simulink model "Flight_Simulation"  (R2021b)
settings: Solver=ode4  StartTime=0.0  StopTime=20  FixedStep=Settings.Simulation.step_size  RelTol=1e-3  EnableMultiTasking=on
undefined symbols (not defined in the file or in its folder): AeroCoeff, Aircraft, ControlGains, dLEF, Environment, F, Light, MIL, Settings, Trim, trim_control, trim_state, trim_thrust
libraries: simulink x19, simulink_extras x14, slpidlib x2, aerolibfltsims x2, aerolibwind2 x1, vrlib x1
(part 3 of 5)

== system Flight_Simulation/Environment_Subsystems/Wind_Input/Bypass for TrimAndLin ==
  note: No time variant wind for TrimAndLin
  Wind_BUS : Inport
  Flag_Settings_BUS : Inport  Port=2
  Bus Creator : BusCreator  Inputs=3
  Bus Selector : BusSelector  OutputSignals=Linearization_Flag,Trim_Flag
  Bypass for TrimAndLin : Switch  Criteria=u2 > Threshold
  Constant : Constant  Value=0
  Constant1 : Constant  Value=0
  Constant2 : Constant  Value=0
  Demux : Demux  Outputs=3
  Logical Operator : Logic  Operator=NOR  AllPortsSameDT=off  OutDataTypeStr=boolean
  Mux1 : Mux  Inputs=3
  Wind_Vel : Outport
  wires:
  Bus Selector/2 -> Logical Operator/2  "<Trim_Flag>"
  Bus Selector/1 -> Logical Operator/1  "<Linearization_Flag>"
  Logical Operator/1 -> Bypass for TrimAndLin/2
  Flag_Settings_BUS/1 -> Bus Selector/1
  Bus Creator/1 -> Wind_Vel/1  "Wind_Vel_UVWe_m/s"
  Demux/1 -> Bus Creator/1  "u_wind_m/s"
  Demux/2 -> Bus Creator/2  "v_wind_m/s"
  Demux/3 -> Bus Creator/3  "w_wind_m/s"
  Bypass for TrimAndLin/1 -> Demux/1
  Wind_BUS/1 -> Bypass for TrimAndLin/1
  Constant1/1 -> Mux1/1  "u_wind_m/s"
  Constant/1 -> Mux1/2  "v_wind_m/s"
  Constant2/1 -> Mux1/3  "w_wind_m/s"
  Mux1/1 -> Bypass for TrimAndLin/3

== system Flight_Simulation/Environment_Subsystems/Wind_Input/Calc_Vel_aero_alpha_beta ==
  Vel_U_V_W_BUS : Inport
  Add : Sum  Inputs=+++
  Atan : Trigonometry  Operator=atan
  Atan1 : Trigonometry  Operator=atan
  Bus Creator : BusCreator  Inputs=3
  Bus Selector : BusSelector  OutputSignals=U_aero_m/s,V_aero_m/s,W_aero_m/s
  Divide : Product  Inputs=*/
  Divide1 : Product  Inputs=*/
  Sqrt : Sqrt  SaturateOnIntegerOverflow=on
  Square : Math  Operator=square  SaturateOnIntegerOverflow=on
  Square1 : Math  Operator=square  SaturateOnIntegerOverflow=on
  Square2 : Math  Operator=square  SaturateOnIntegerOverflow=on
  Vel_aero_alpha_beta_BUS : Outport
  wires:
  Vel_U_V_W_BUS/1 -> Bus Selector/1
  Bus Creator/1 -> Vel_aero_alpha_beta_BUS/1  "Vel_aero_V_alpha_beta"
  Sqrt/1 -> Bus Creator/1  "v_m/s"
  Atan/1 -> Bus Creator/2  "alpha_rad"
  Atan1/1 -> Bus Creator/3  "beta_rad"
  Bus Selector/1 -> Divide1/2, Divide/2, Square/1  "<U_aero_m/s>"
  Bus Selector/2 -> Square1/1, Divide1/1  "<V_aero_m/s>"
  Bus Selector/3 -> Divide/1, Square2/1  "<W_aero_m/s>"
  Add/1 -> Sqrt/1
  Square2/1 -> Add/3
  Square1/1 -> Add/2
  Square/1 -> Add/1
  Divide/1 -> Atan/1
  Divide1/1 -> Atan1/1

== system Flight_Simulation/Environment_Subsystems/Wind_Model/Gust_model_(1-cos) ==
  note: To stop the "distance traveled
      | through the gust counter"
  Atmosphere_BUS : Inport
  FlightProfileAlleviationFactor_Fg : Inport  Port=2
  altitude_m : Inport  Port=3
  v_m/s : Inport  Port=4
  1-cos_gust_flg : Step  Time=Environment.gust.steptimes  After=Environment.gust.flags  SampleTime=0
  Abs1 : Abs
  Distance traveled through the gust : Subsystem
  Gust parameters : Subsystem
  Gust velocity (1-cos) : Subsystem
      mask Display: image('1-cos-gust.png'); % Use "Edit Image" on toolstrip to change.
  Sum1 : Sum  Inputs=|+-
  reset flags after gust : Subsystem
  u_wind_m/s : Outport
  v_wind_m/s : Outport  Port=2
  w_wind_m/s : Outport  Port=3
  wires:
  Sum1/1 -> Distance traveled through the gust/2(gust_flgs)  "gust_flgs"
  reset flags after gust/1(reset_flgs) -> Sum1/2
  1-cos_gust_flg/1 -> Abs1/1, Gust velocity (1-cos)/4(Sign_Input)  "Sign_carry"
  altitude_m/1 -> Gust parameters/3(altitude)
  Gust parameters/1(gust_gradient_length) -> Gust velocity (1-cos)/1(gust_gradient_length)
  Abs1/1 -> Sum1/1
  Gust parameters/2(gust_amplitudes) -> Gust velocity (1-cos)/2(gust_amplitudes)
  Distance traveled through the gust/1(distance_traveled) -> Gust velocity (1-cos)/3(distance_traveled)  "distance_traveled_xyz"
  Gust velocity (1-cos)/2(Gust_Vel_V_m/s) -> reset flags after gust/2(gust_v), v_wind_m/s/1  "v_wind_m/s"
  v_m/s/1 -> Distance traveled through the gust/1(v_m/s)
  FlightProfileAlleviationFactor_Fg/1 -> Gust parameters/2(F_g)
  Gust velocity (1-cos)/1(Gust_Vel_U_m/s) -> reset flags after gust/1(gust_u), u_wind_m/s/1  "u_wind_m/s"
  Gust velocity (1-cos)/3(Gust_Vel_W_m/s) -> reset flags after gust/3(gust_w), w_wind_m/s/1  "w_wind_m/s"
  Atmosphere_BUS/1 -> Gust parameters/1(Atmosphere_BUS)

== system Flight_Simulation/Non-linear_Plant/6DOF_Equations/Acceleration_nx_ny_nz_Calculation ==
  Vel_U_V_W_dot_BUS : Inport
  States_BUS : Inport  Port=2
  Gravity_BUS : Inport  Port=3
  Bus Creator : BusCreator  Inputs=3
  nx_cg : Subsystem
  ny_cg : Subsystem
  nz_cg : Subsystem
  Acc_nx_ny_nz_BUS : Outport
  wires:
  States_BUS/1 -> nx_cg/1(States_BUS), nz_cg/1(States_BUS), ny_cg/1(States_BUS)
  Vel_U_V_W_dot_BUS/1 -> nx_cg/2(Vel_U_V_W_dot_BUS), nz_cg/2(Vel_U_V_W_dot_BUS), ny_cg/2(Vel_U_V_W_dot_BUS)
  Gravity_BUS/1 -> nx_cg/3(Gravity), nz_cg/3(Gravity), ny_cg/3(Gravity)
  Bus Creator/1 -> Acc_nx_ny_nz_BUS/1
  nx_cg/1(n_x_cg) -> Bus Creator/1
  ny_cg/1(n_y_cg) -> Bus Creator/2
  nz_cg/1(n_z_cg) -> Bus Creator/3

== system Flight_Simulation/Non-linear_Plant/6DOF_Equations/Attitude_Differential_Equations ==
  States_BUS : Inport
  Bus Creator : BusCreator  Inputs=3
  Bus Selector : BusSelector  OutputSignals=Angles_phi_theta_psi,Rates_p_q_r
  Bus Selector1 : BusSelector  OutputSignals=phi_rad,theta_rad,psi_rad
  Bus Selector2 : BusSelector  OutputSignals=p_rad/s,q_rad/s,r_rad/s
  phi_dot : Subsystem
  psi_dot : Subsystem
  theta_dot : Subsystem
  Attitude_dot_BUS : Outport
  wires:
  States_BUS/1 -> Bus Selector/1
  Bus Selector/1 -> Bus Selector1/1  "<Angles_phi_theta_psi>"
  Bus Selector/2 -> Bus Selector2/1  "<Rates_p_q_r>"
  Bus Creator/1 -> Attitude_dot_BUS/1  "Angles_dot_phi_theta_psi"
  Bus Selector1/1 -> phi_dot/1(phi), theta_dot/1(phi), psi_dot/1(phi)  "<phi_rad>"
  Bus Selector1/2 -> phi_dot/2(theta), theta_dot/2(theta), psi_dot/2(theta)  "<theta_rad>"
  Bus Selector1/3 -> phi_dot/3(psi), psi_dot/3(psi), theta_dot/3(psi)  "<psi_rad>"
  Bus Selector2/1 -> phi_dot/4(p), psi_dot/4(p), theta_dot/4(p)  "<p_rad/s>"
  Bus Selector2/2 -> phi_dot/5(q), psi_dot/5(q), theta_dot/5(q)  "<q_rad/s>"
  Bus Selector2/3 -> phi_dot/6(r), psi_dot/6(r), theta_dot/6(r)  "<r_rad/s>"
  phi_dot/1(phi_dot_rad/s) -> Bus Creator/1
  theta_dot/1(theta_dot_rad/s) -> Bus Creator/2
  psi_dot/1(psi_dot_rad/s) -> Bus Creator/3

== system Flight_Simulation/Non-linear_Plant/6DOF_Equations/Position_Differential_Equations ==
  Earth_Model_BUS : Inport
  States_BUS : Inport  Port=2
  Bus Creator : BusCreator  Inputs=3
  Bus Creator2 : BusCreator  Inputs=2
  Bus Selector : BusSelector  OutputSignals=Angles_phi_theta_psi
  Bus Selector1 : BusSelector  OutputSignals=U_m/s,V_m/s,W_m/s
  Bus Selector2 : BusSelector  OutputSignals=Pos_WGS84
  Bus Selector3 : BusSelector  OutputSignals=phi_rad,theta_rad,psi_rad
  Bus Selector4 : BusSelector  OutputSignals=Vel_U_V_W_body
  Calculate_alt_position_dot1 : Subsystem
  Calculate_east_position_dot : Subsystem
  Calculate_north_position_dot : Subsystem
  Position_dot_WGS84 : Subsystem
  Position_dot_BUS : Outport
  wires:
  Bus Creator/1 -> Bus Creator2/1  "Position_dot_north_east_alt"
  Bus Selector/1 -> Bus Selector3/1  "<Angles_phi_theta_psi>"
  Bus Selector1/1 -> Calculate_north_position_dot/1(U), Calculate_east_position_dot/1(U), Calculate_alt_position_dot1/1(U)  "<U_m/s>"
  Bus Selector1/2 -> Calculate_north_position_dot/2(V), Calculate_alt_position_dot1/2(V), Calculate_east_position_dot/2(V)  "<V_m/s>"
  Bus Selector1/3 -> Calculate_north_position_dot/3(W), Calculate_alt_position_dot1/3(W), Calculate_east_position_dot/3(W)  "<W_m/s>"
  Bus Selector3/1 -> Calculate_north_position_dot/4(phi), Calculate_alt_position_dot1/4(phi), Calculate_east_position_dot/4(phi)  "<phi_rad>"
  Bus Selector3/2 -> Calculate_alt_position_dot1/5(theta), Calculate_east_position_dot/5(theta), Calculate_north_position_dot/5(theta)  "<theta_rad>"
  Bus Selector3/3 -> Calculate_alt_position_dot1/6(psi), Calculate_east_position_dot/6(psi), Calculate_north_position_dot/6(psi)  "<psi_rad>"
  Calculate_north_position_dot/1(north_pos_dot) -> Position_dot_WGS84/1(U_earth), Bus Creator/1
  Calculate_east_position_dot/1(east_pos_dot) -> Position_dot_WGS84/2(V_earth), Bus Creator/2
  Calculate_alt_position_dot1/1(alt_dot) -> Position_dot_WGS84/3(alt_dot), Bus Creator/3
  Earth_Model_BUS/1 -> Position_dot_WGS84/5(Earth_Model_BUS)
  Position_dot_WGS84/1(Pos_WGS84_dot_BUS) -> Bus Creator2/2
  Bus Creator2/1 -> Position_dot_BUS/1  "Position_dot_BUS"
  Bus Selector2/1 -> Position_dot_WGS84/4(Pos_WGS84)  "<Pos_WGS84>"
  States_BUS/1 -> Bus Selector4/1, Bus Selector2/1, Bus Selector/1
  Bus Selector4/1 -> Bus Selector1/1  "<Vel_U_V_W_body>"

== system Flight_Simulation/Non-linear_Plant/6DOF_Equations/Rotation_Differential_Equation ==
  Aircraft_Constants_BUS : Inport
  Engine_BUS : Inport  Port=2
  States_BUS : Inport  Port=3
  Moments_total_BUS : Inport  Port=4
  Bus Creator1 : BusCreator  Inputs=3
  Inertia_Denominator_Calculation : Subsystem
  p_dot_Calculation : Subsystem
  q_dot_Calculation : Subsystem
  r_dot_Calculation : Subsystem
  Rates_dot_p_q_r : Outport
  wires:
  Aircraft_Constants_BUS/1 -> r_dot_Calculation/3(Aircraft_Constants_BUS), p_dot_Calculation/2(Aircraft_Constants_BUS), q_dot_Calculation/2(Aircraft_Constants_BUS), Inertia_Denominator_Calculation/1(Aircraft_Constants_BUS)
  States_BUS/1 -> r_dot_Calculation/2(States_BUS), p_dot_Calculation/3(States_BUS), q_dot_Calculation/1(States_BUS)
  Inertia_Denominator_Calculation/1(Inertia_Denominator) -> r_dot_Calculation/1(Inertia_Denominator), p_dot_Calculation/4(Inertia_Denominator)
  Moments_total_BUS/1 -> r_dot_Calculation/4(Moments_total_BUS), p_dot_Calculation/1(Moments_total_BUS), q_dot_Calculation/3(Moments_total_BUS)  "Moments_total_BUS"
  p_dot_Calculation/1(p_dot) -> Bus Creator1/1
  q_dot_Calculation/1(q_dot) -> Bus Creator1/2
  Bus Creator1/1 -> Rates_dot_p_q_r/1  "Rates_dot_p_q_r"
  r_dot_Calculation/1(r_dot) -> Bus Creator1/3
  Engine_BUS/1 -> q_dot_Calculation/4(Engine_BUS)

== system Flight_Simulation/Non-linear_Plant/6DOF_Equations/Translation_UVW_Differential_Equations ==
  States_BUS : Inport
  Forces_total_BUS : Inport  Port=2
  Engine_BUS : Inport  Port=3
  Aircraft_Constants_BUS : Inport  Port=4
  Gravity_BUS : Inport  Port=5
  Bus Creator : BusCreator  Inputs=3
  U_dot : Subsystem
  V_dot : Subsystem
  W_dot : Subsystem
  Vel_U_V_W_body_dot_BUS : Outport
  wires:
  Bus Creator/1 -> Vel_U_V_W_body_dot_BUS/1  "Vel_U_V_W_body_dot_BUS"
  U_dot/1(U_dot) -> Bus Creator/1
  States_BUS/1 -> U_dot/1(States_BUS), V_dot/1(States_BUS), W_dot/1(States_BUS)
  Forces_total_BUS/1 -> W_dot/2(Force_Coeff_BUS), U_dot/2(Forces_total_BUS), V_dot/2(Forces_total_BUS)
  Aircraft_Constants_BUS/1 -> U_dot/3(Aircraft_Constants_BUS), W_dot/3(Aircraft_Constants_BUS), V_dot/3(Aircraft_Constants_BUS1)
  Gravity_BUS/1 -> W_dot/4(Gravity_BUS), V_dot/4(Gravity_BUS), U_dot/4(Gravity_BUS)
  Engine_BUS/1 -> U_dot/5(Engine_BUS)
  V_dot/1(V_dot) -> Bus Creator/2
  W_dot/1(W_dot) -> Bus Creator/3

== system Flight_Simulation/Non-linear_Plant/Actuator_Models/Aileron Actuator ==
  note: Mustn't change the name of integrator representing the position
      | xxx_pos_int as this will interfere with the trim and lin routine
  Aileron_cmd_deg : Inport
  Control_Surface_Const_BUS : Inport  Port=2
  Aileron_init_deg : Inport  Port=3
  Ail_pos_int : Integrator  InitialConditionSource=external  InitialCondition=trim_control(2)  UpperSaturationLimit=21.5  LowerSaturationLimit=-21.5
  Bus Selector : BusSelector  OutputSignals=Aileron_BUS.Ail_pos_max_deg,Aileron_BUS.Ail_pos_min_deg,Aileron_BUS.Ail_rate_max_degPs,Aileron_BUS.Ail_rate_min_degPs,Aileron_BUS.Ail_lag_s
  Command Saturation : simulink/Discontinuities/Saturation Dynamic  OutMin=[]  OutMax=[]  OutDataTypeStr=Inherit: Same as second input  OutDataType=fixdt(1, 16)  OutScaling=2^-10  DoSatur=off
  Divide : Product  Inputs=/*
  Rate Saturation : simulink/Discontinuities/Saturation Dynamic  OutMin=[]  OutMax=[]  OutDataTypeStr=Inherit: Same as second input  OutDataType=fixdt(1, 16)  OutScaling=2^-10  DoSatur=off
  Sum : Sum  Inputs=|+-  InputSameDT=on  SaturateOnIntegerOverflow=on  OutDataTypeStr=Inherit: Same as first input
  Aileron_act_deg : Outport
  wires:
  Rate Saturation/1 -> Ail_pos_int/1
  Aileron_cmd_deg/1 -> Command Saturation/2
  Aileron_init_deg/1 -> Ail_pos_int/2
  Bus Selector/3 -> Rate Saturation/1  "<Ail_rate_max_degPs>"
  Bus Selector/5 -> Divide/1  "<Ail_lag_s>"
  Bus Selector/4 -> Rate Saturation/3  "<Ail_rate_min_degPs>"
  Control_Surface_Const_BUS/1 -> Bus Selector/1
  Divide/1 -> Rate Saturation/2
  Bus Selector/1 -> Command Saturation/1  "<Ail_pos_max_deg>"
  Bus Selector/2 -> Command Saturation/3  "<Ail_pos_min_deg>"
  Command Saturation/1 -> Sum/1
  Sum/1 -> Divide/2
  Ail_pos_int/1 -> Aileron_act_deg/1, Sum/2

== system Flight_Simulation/Non-linear_Plant/Actuator_Models/Elevator Actuator ==
  note: Mustn't change the name of integrator representing the position
      | xxx_pos_int as this will interfere with the trim and lin routine
  Elevator_cmd_deg : Inport
  Control_Surface_Const_BUS : Inport  Port=2
  Elevator_init_deg : Inport  Port=3
  Bus Selector : BusSelector  OutputSignals=Elevator_BUS.Elev_pos_max_deg,Elevator_BUS.Elev_pos_min_deg,Elevator_BUS.Elev_rate_max_degPs,Elevator_BUS.Elev_rate_min_degPs,Elevator_BUS.Elev_lag_s
  Command Saturation : simulink/Discontinuities/Saturation Dynamic  OutMin=[]  OutMax=[]  OutDataTypeStr=Inherit: Same as second input  OutDataType=fixdt(1, 16)  OutScaling=2^-10  DoSatur=off
  Divide : Product  Inputs=/*
  Elev_pos_int : Integrator  InitialConditionSource=external  InitialCondition=trim_control(1)  UpperSaturationLimit=25  LowerSaturationLimit=-25
  Rate Saturation : simulink/Discontinuities/Saturation Dynamic  OutMin=[]  OutMax=[]  OutDataTypeStr=Inherit: Same as second input  OutDataType=fixdt(1, 16)  OutScaling=2^-10  DoSatur=off
  Sum : Sum  Inputs=|+-  InputSameDT=on  SaturateOnIntegerOverflow=on  OutDataTypeStr=Inherit: Same as first input
  Elevator_act_deg : Outport
  wires:
  Rate Saturation/1 -> Elev_pos_int/1
  Divide/1 -> Rate Saturation/2
  Sum/1 -> Divide/2
  Command Saturation/1 -> Sum/1
  Elevator_cmd_deg/1 -> Command Saturation/2
  Elevator_init_deg/1 -> Elev_pos_int/2
  Control_Surface_Const_BUS/1 -> Bus Selector/1
  Bus Selector/1 -> Command Saturation/1  "<Elev_pos_max_deg>"
  Bus Selector/2 -> Command Saturation/3  "<Elev_pos_min_deg>"
  Bus Selector/3 -> Rate Saturation/1  "<Elev_rate_max_degPs>"
  Bus Selector/4 -> Rate Saturation/3  "<Elev_rate_min_degPs>"
  Bus Selector/5 -> Divide/1  "<Elev_lag_s>"
  Elev_pos_int/1 -> Elevator_act_deg/1, Sum/2

== system Flight_Simulation/Non-linear_Plant/Actuator_Models/Leading Edge Flap ==
  note: initial state was:
      | -trim_state(8)*180/pi /// -alpha*180/pi
      |
      | set to 0 now, cause leading edge flap is not in use
      | change that to make the system more efficient
  note: see NASA Technical Paper 1538, p34
  note: Initialize LF_state with -alpha0 value in degrees!!!!
  Atmosphere_BUS : Inport
  States_BUS : Inport  Port=2
  Bus Selector1 : BusSelector  OutputSignals=alpha_rad
  Bus Selector2 : BusSelector  OutputSignals=Vel_aero_V_alpha_beta
  Bus Selector3 : BusSelector  OutputSignals=q_bar_Pa,p_static_Pa
  Divide : Product  Inputs=*/
  Gain : Gain  Gain=2  SaturateOnIntegerOverflow=on  OutDataTypeStr=Inherit: Same as input  ParamDataTypeStr=Inherit: Same as input
  Gain1 : Gain  Gain=7.25  SaturateOnIntegerOverflow=on  OutDataTypeStr=Inherit: Same as input  ParamDataTypeStr=Inherit: Same as input
  Gain2 : Gain  Gain=1.38  SaturateOnIntegerOverflow=on  OutDataTypeStr=Inherit: Same as input  ParamDataTypeStr=Inherit: Same as input
  LEF Actuator : Subsystem
  LEF deflection : ToWorkspace  Commented=on  VariableName=d_LF  SampleTime=-1
      settings: Decimation=100
  LF_state : Integrator
  Sum : Sum  Inputs=-|+|+  InputSameDT=on  SaturateOnIntegerOverflow=on  OutDataTypeStr=Inherit: Same as first input
  Sum1 : Sum  Inputs=|+-  InputSameDT=on  SaturateOnIntegerOverflow=on  OutDataTypeStr=Inherit: Same as first input
  Sum2 : Sum  Inputs=++|  InputSameDT=on  SaturateOnIntegerOverflow=on  OutDataTypeStr=Inherit: Same as first input
  coeff1 : Constant  Value=1.45
  r2d1 : Gain  Gain=180/pi  SaturateOnIntegerOverflow=on  OutDataTypeStr=Inherit: Same as input  ParamDataTypeStr=Inherit: Same as input
  r2d6 : Gain  Gain=9.05  SaturateOnIntegerOverflow=on  OutDataTypeStr=Inherit: Same as input  ParamDataTypeStr=Inherit: Same as input
  LE_Flap_deg : Outport
  wires:
  LEF Actuator/1(Out1) -> LEF deflection/1, LE_Flap_deg/1
  Sum/1 -> LEF Actuator/1(In1)
  States_BUS/1 -> Bus Selector2/1
  Sum1/1 -> Gain1/1
  Gain1/1 -> LF_state/1
  Gain/1 -> Sum2/1
  Gain2/1 -> Sum/2
  coeff1/1 -> Sum/3
  Sum2/1 -> Sum1/2, Gain2/1
  LF_state/1 -> Sum2/2
  r2d1/1 -> Sum1/1, Gain/1  "alpha"
  Divide/1 -> r2d6/1
  r2d6/1 -> Sum/1
  Bus Selector2/1 -> Bus Selector1/1  "<Vel_aero_V_alpha_beta>"
  Bus Selector1/1 -> r2d1/1  "<alpha_rad>"
  Atmosphere_BUS/1 -> Bus Selector3/1
  Bus Selector3/1 -> Divide/1  "<q_bar_Pa>"
  Bus Selector3/2 -> Divide/2  "<p_static_Pa>"

== system Flight_Simulation/Non-linear_Plant/Actuator_Models/Rudder Actuator ==
  note: Mustn't change the name of integrator representing the position
      | xxx_pos_int as this will interfere with the trim and lin routine
  Rudder_cmd_deg : Inport
  Control_Surface_Const_BUS : Inport  Port=2
  Rudder_init_deg : Inport  Port=3
  Bus Selector : BusSelector  OutputSignals=Rudder_BUS.Rud_pos_max_deg,Rudder_BUS.Rud_pos_min_deg,Rudder_BUS.Rud_rate_max_degPs,Rudder_BUS.Rud_rate_min_degPs,Rudder_BUS.Rud_lag_s
  Command Saturation : simulink/Discontinuities/Saturation Dynamic  OutMin=[]  OutMax=[]  OutDataTypeStr=Inherit: Same as second input  OutDataType=fixdt(1, 16)  OutScaling=2^-10  DoSatur=off
  Divide : Product  Inputs=/*
  Rate Saturation : simulink/Discontinuities/Saturation Dynamic  OutMin=[]  OutMax=[]  OutDataTypeStr=Inherit: Same as second input  OutDataType=fixdt(1, 16)  OutScaling=2^-10  DoSatur=off
  Rud_pos_int : Integrator  InitialConditionSource=external  InitialCondition=trim_control(3)  UpperSaturationLimit=30  LowerSaturationLimit=-30
  Sum : Sum  Inputs=|+-  InputSameDT=on  SaturateOnIntegerOverflow=on  OutDataTypeStr=Inherit: Same as first input
  Rudder_act_deg : Outport
  wires:
  Rate Saturation/1 -> Rud_pos_int/1
  Rudder_cmd_deg/1 -> Command Saturation/2
  Rudder_init_deg/1 -> Rud_pos_int/2
  Bus Selector/3 -> Rate Saturation/1  "<Rud_rate_max_degPs>"
  Bus Selector/5 -> Divide/1  "<Rud_lag_s>"
  Bus Selector/4 -> Rate Saturation/3  "<Rud_rate_min_degPs>"
  Control_Surface_Const_BUS/1 -> Bus Selector/1
  Divide/1 -> Rate Saturation/2
  Bus Selector/1 -> Command Saturation/1  "<Rud_pos_max_deg>"
  Bus Selector/2 -> Command Saturation/3  "<Rud_pos_min_deg>"
  Command Saturation/1 -> Sum/1
  Sum/1 -> Divide/2
  Rud_pos_int/1 -> Rudder_act_deg/1, Sum/2

== system Flight_Simulation/Non-linear_Plant/Aerodynamic_Modul/Aero_Coefficients ==
  note: F16:
      | the gridding right now is arkward ... for Force-control-Coeff! - especially Elevator
      | the c code has some issues ... first break point is +-12deg
      | it never hits the boundaries in any case (alpha, eta) just for beta but there the extrapolation is bullshit
      | so the c code will be fixed so that the results work and fit the simulink case
  Aircraft_Constant_BUS : Inport
  Atmosphere_BUS : Inport  Port=2
  Controls_BUS : Inport  Port=3
  Engine_BUS : Inport  Port=4
  States_BUS : Inport  Port=5
  Controls unit preparation : Subsystem
  Force_Coefficients : Subsystem
  Moment_Coefficients : Subsystem
  alpha beta unit preparation : Subsystem
  Force_Coeff_BUS : Outport
  Moment_Coeff_BUS : Outport  Port=2
  wires:
  Controls_BUS/1 -> Controls unit preparation/1(Controls_BUS)
  Aircraft_Constant_BUS/1 -> Moment_Coefficients/4(Aircraft_Constant_BUS), Force_Coefficients/4(Aircraft_Constant_BUS)
  States_BUS/1 -> Moment_Coefficients/2(States_BUS), Force_Coefficients/2(States_BUS), alpha beta unit preparation/1(States_BUS)
  alpha beta unit preparation/1(alpha_beta) -> Moment_Coefficients/3(alpha_beta), Force_Coefficients/3(alpha_beta)
  Engine_BUS/1 -> Moment_Coefficients/6(Engine_BUS), Force_Coefficients/6(Engine_BUS)
  Controls unit preparation/1(prep_Controls_BUS) -> Moment_Coefficients/5(prep_Controls_BUS), Force_Coefficients/5(prep_Controls_BUS)
  Force_Coefficients/1(Force_Coeff_BUS) -> Force_Coeff_BUS/1, Moment_Coefficients/1(Force_Coefficients)
  Moment_Coefficients/1(Moment_Coeff_BUS) -> Moment_Coeff_BUS/1
  Atmosphere_BUS/1 -> Force_Coefficients/1(Atmosphere_BUS)

== system Flight_Simulation/Non-linear_Plant/Aerodynamic_Modul/States with Wind ==
  States_BUS : Inport
  Vel_aero_BUS : Inport  Port=2
  Bus Creator : BusCreator  Inputs=6
  Bus Selector : BusSelector  OutputSignals=Position_north_east_alt,Angles_phi_theta_psi,Rates_p_q_r,Pos_WGS84
  Bus Selector1 : BusSelector  OutputSignals=Vel_aero_V_alpha_beta,Vel_U_V_W_aero
  New_States_BUS : Outport
  wires:
  Vel_aero_BUS/1 -> Bus Selector1/1
  Bus Selector/1 -> Bus Creator/1  "<Position_north_east_alt>"
  States_BUS/1 -> Bus Selector/1
  Bus Selector/2 -> Bus Creator/2  "<Angles_phi_theta_psi>"
  Bus Creator/1 -> New_States_BUS/1
  Bus Selector/3 -> Bus Creator/3  "<Rates_p_q_r>"
  Bus Selector/4 -> Bus Creator/4  "<Pos_WGS84>"
  Bus Selector1/1 -> Bus Creator/5  "<Vel_aero_V_alpha_beta>"
  Bus Selector1/2 -> Bus Creator/6  "<Vel_U_V_W_aero>"

== system Flight_Simulation/Non-linear_Plant/Aerodynamic_Modul/Total Aero Forces ==
  Atmosphere_BUS : Inport
  Aircraft_Constants_BUS : Inport  Port=2
  Force_Coeff_BUS : Inport  Port=3
  Bus Creator : BusCreator  Inputs=3
  Bus Selector10 : BusSelector  OutputSignals=C_x_total,C_y_total,C_z_total
  Bus Selector6 : BusSelector  OutputSignals=q_bar_Pa
  Bus Selector8 : BusSelector  OutputSignals=Wing_Dimension_BUS.WingArea_m^2
  Product1 : Product  Inputs=3
  Product2 : Product  Inputs=3
  Product3 : Product  Inputs=3
  Forces_total_BUS : Outport
  wires:
  Product3/1 -> Bus Creator/3  "Z_total"
  Bus Selector6/1 -> Product2/3, Product1/3, Product3/3  "<q_bar_Pa>"
  Atmosphere_BUS/1 -> Bus Selector6/1
  Force_Coeff_BUS/1 -> Bus Selector10/1
  Bus Selector8/1 -> Product2/2, Product1/2, Product3/2  "<WingArea_m^2>"
  Aircraft_Constants_BUS/1 -> Bus Selector8/1
  Bus Selector10/1 -> Product2/1  "<C_x_total>"
  Bus Selector10/2 -> Product1/1  "<C_y_total>"
  Bus Selector10/3 -> Product3/1  "<C_z_total>"
  Product2/1 -> Bus Creator/1  "X_total"
  Product1/1 -> Bus Creator/2  "Y_total"
  Bus Creator/1 -> Forces_total_BUS/1  "Forces_total_BUS"

== system Flight_Simulation/Non-linear_Plant/Aerodynamic_Modul/Total Aero Moments ==
  Atmosphere_BUS : Inport
  Aircraft_Constants_BUS : Inport  Port=2
  Moment_Coeff_BUS : Inport  Port=3
  Bus Creator : BusCreator  Inputs=3
  L_total_Calculation : Subsystem
  M_total_Calculation : Subsystem
  N_total_Calculation : Subsystem
  Moments_total_BUS : Outport
  wires:
  Bus Creator/1 -> Moments_total_BUS/1  "Moments_total_BUS"
  Aircraft_Constants_BUS/1 -> L_total_Calculation/2(Aircraft_Constants_BUS), M_total_Calculation/2(Aircraft_Constants_BUS), N_total_Calculation/2(Aircraft_Constants_BUS)
  L_total_Calculation/1(L_total) -> Bus Creator/1
  Atmosphere_BUS/1 -> N_total_Calculation/1(Atmosphere_BUS), L_total_Calculation/1(Atmosphere_BUS), M_total_Calculation/1(Atmosphere_BUS)
  Moment_Coeff_BUS/1 -> L_total_Calculation/3(Moment_Coeff_BUS), M_total_Calculation/3(Moment_Coeff_BUS), N_total_Calculation/3(Moment_Coeff_BUS)
  N_total_Calculation/1(N_total) -> Bus Creator/3
  M_total_Calculation/1(M_total) -> Bus Creator/2

== system Flight_Simulation/Non-linear_Plant/Aerodynamic_Modul/Wind to body axis rotation ==
  note: Flags to turn transformation on/off
      | - set in InitAeroCoeff script
  Forces_wind : Inport
  Moments_wind : Inport  Port=2
  States_BUS : Inport  Port=3
  Bus Creator : BusCreator  Inputs=3
  Bus Creator1 : BusCreator  Inputs=3
  Bus Selector : BusSelector  OutputSignals=X_total,Y_total,Z_total
  Bus Selector1 : BusSelector  OutputSignals=L_total,M_total,N_total
  Bus Selector2 : BusSelector  OutputSignals=Vel_aero_V_alpha_beta.alpha_rad,Vel_aero_V_alpha_beta.beta_rad
  Gain : Gain  Gain=AeroCoeff.alpha_wind
  Gain1 : Gain  Gain=AeroCoeff.beta_wind
  Wind to body axis rotation : MATLAB Function  TreatAsAtomicUnit=on
  Forces_body : Outport
  Moments_body : Outport  Port=2
  wires:
  Wind to body axis rotation/4(Lb) -> Bus Creator1/1  "L_total"
  Bus Selector1/2 -> Wind to body axis rotation/5(Mw)  "<M_total>"
  Wind to body axis rotation/1(Xb) -> Bus Creator/1  "X_total"
  Bus Selector/3 -> Wind to body axis rotation/3(Zw)  "<Z_total>"
  Bus Selector/1 -> Wind to body axis rotation/1(Xw)  "<X_total>"
  Forces_wind/1 -> Bus Selector/1
  Bus Creator1/1 -> Moments_body/1  "Moments_total_BUS"
  Bus Selector1/1 -> Wind to body axis rotation/4(Lw)  "<L_total>"
  Wind to body axis rotation/3(Zb) -> Bus Creator/3  "Z_total"
  Bus Selector2/1 -> Gain/1  "<alpha_rad>"
  Wind to body axis rotation/2(Yb) -> Bus Creator/2  "Y_total"
  Wind to body axis rotation/5(Mb) -> Bus Creator1/2  "M_total"
  Bus Selector1/3 -> Wind to body axis rotation/6(Nw)  "<N_total>"
  Bus Selector/2 -> Wind to body axis rotation/2(Yw)  "<Y_total>"
  Bus Selector2/2 -> Gain1/1  "<beta_rad>"
  Wind to body axis rotation/6(Nb) -> Bus Creator1/3  "N_total"
  Gain/1 -> Wind to body axis rotation/7(alfa_rad)
  Gain1/1 -> Wind to body axis rotation/8(beta_rad)
  States_BUS/1 -> Bus Selector2/1
  Moments_wind/1 -> Bus Selector1/1
  Bus Creator/1 -> Forces_body/1  "Forces_total_BUS"

== system Flight_Simulation/Non-linear_Plant/Engine_Model/Propeller CT Calculation ==
  Thrust_cmd_N : Inport
  q_bar_Pa : Inport  Port=2
  Propeler_S_m^2 : Inport  Port=3
  Bus Selector : BusSelector  OutputSignals=Propeler_S_m^2
  Constant : Constant
  Ct : Product  Inputs=*//  RndMeth=Zero  SaturateOnIntegerOverflow=on
  Product : Product
  avoid 0 division : Switch  Criteria=u2 > Threshold
  multiply 0 if S_prop = 0 : Switch  Criteria=u2 > Threshold
  CT : Outport
  wires:
  q_bar_Pa/1 -> Ct/2
  Ct/1 -> Product/1  "CT"
  Thrust_cmd_N/1 -> Ct/1
  Bus Selector/1 -> avoid 0 division/1, multiply 0 if S_prop = 0/3, multiply 0 if S_prop = 0/2, avoid 0 division/2  "<Propeler_S_m^2>"
  avoid 0 division/1 -> Ct/3
  Constant/1 -> avoid 0 division/3, multiply 0 if S_prop = 0/1
  Product/1 -> CT/1  "CT"
  multiply 0 if S_prop = 0/1 -> Product/2
  Propeler_S_m^2/1 -> Bus Selector/1

== system Flight_Simulation/Non-linear_Plant/Engine_Model/Thrust Model ==
  note: Mustn't change the name of integrator representing the position
      | xxx_pos_int as this will interfere with the trim and lin routine
  Thrust_cmd_N : Inport
  Thrust_init_N : Inport  Port=2
  Aircraft_Constants_BUS : Inport  Port=3
  Bus Selector : BusSelector  OutputSignals=thrust_max,thrust_min,thrust_rate_max,thrust_rate_min,thrust_lag
  Command Saturation : simulink/Discontinuities/Saturation Dynamic  OutMin=[]  OutMax=[]  OutDataTypeStr=Inherit: Same as second input  OutDataType=fixdt(1, 16)  OutScaling=2^-10  DoSatur=off
  Divide : Product  Inputs=/*
  Rate Saturation : simulink/Discontinuities/Saturation Dynamic  OutMin=[]  OutMax=[]  OutDataTypeStr=Inherit: Same as second input  OutDataType=fixdt(1, 16)  OutScaling=2^-10  DoSatur=off
  Sum : Sum  Inputs=|+-  InputSameDT=on  SaturateOnIntegerOverflow=on  OutDataTypeStr=Inherit: Same as first input
  Thrust_pos_int : Integrator  InitialConditionSource=external  InitialCondition=trim_thrust  UpperSaturationLimit=30  LowerSaturationLimit=-30
  Thrust_act_N : Outport
  wires:
  Thrust_pos_int/1 -> Sum/2, Thrust_act_N/1
  Rate Saturation/1 -> Thrust_pos_int/1
  Divide/1 -> Rate Saturation/2
  Sum/1 -> Divide/2
  Command Saturation/1 -> Sum/1
  Thrust_cmd_N/1 -> Command Saturation/2
  Thrust_init_N/1 -> Thrust_pos_int/2
  Aircraft_Constants_BUS/1 -> Bus Selector/1
  Bus Selector/1 -> Command Saturation/1  "<thrust_max>"
  Bus Selector/2 -> Command Saturation/3  "<thrust_min>"
  Bus Selector/3 -> Rate Saturation/1  "<thrust_rate_max>"
  Bus Selector/4 -> Rate Saturation/3  "<thrust_rate_min>"
  Bus Selector/5 -> Divide/1  "<thrust_lag>"

== system Flight_Simulation/State_Integration_pure_simulink/Vel_aero_dot_Calculation/Vel_aero_dot_total ==
  States_BUS : Inport
  Vel_U_V_W_BUS : Inport  Port=2
  Vel_U_V_W_dot_BUS : Inport  Port=3
  Bus Selector : BusSelector  OutputSignals=Vel_aero_V_alpha_beta
  Bus Selector1 : BusSelector  OutputSignals=v_m/s
  Bus Selector2 : BusSelector  OutputSignals=U_dot,V_dot,W_dot
  Bus Selector3 : BusSelector  OutputSignals=U,V,W
  Divide : Product  Inputs=/*
  Product : Product
  Product1 : Product
  Product2 : Product
  Sum : Sum  Inputs=3
  V_aero_tot_dot : Outport
  wires:
  Vel_U_V_W_BUS/1 -> Bus Selector3/1
  Bus Selector/1 -> Bus Selector1/1  "<Vel_aero_V_alpha_beta>"
  Divide/1 -> V_aero_tot_dot/1  "v_dot_m/s^2"
  Product/1 -> Sum/1
  Product2/1 -> Sum/3
  Bus Selector2/1 -> Product/2  "<U_dot>"
  Bus Selector3/2 -> Product1/1  "<V>"
  States_BUS/1 -> Bus Selector/1
  Product1/1 -> Sum/2
  Sum/1 -> Divide/2
  Bus Selector2/3 -> Product2/2  "<W_dot>"
  Bus Selector2/2 -> Product1/2  "<V_dot>"
  Bus Selector1/1 -> Divide/1  "<v_m/s>"
  Bus Selector3/1 -> Product/1  "<U>"
  Bus Selector3/3 -> Product2/1  "<W>"
  Vel_U_V_W_dot_BUS/1 -> Bus Selector2/1

== system Flight_Simulation/State_Integration_pure_simulink/Vel_aero_dot_Calculation/alpha_aero_dot ==
  States_BUS : Inport
  Vel_U_V_W_BUS : Inport  Port=2
  Vel_U_V_W_dot_BUS : Inport  Port=3
  Bus Selector2 : BusSelector  OutputSignals=U_dot,W_dot
  Bus Selector3 : BusSelector  OutputSignals=U,W
  Divide : Product  Inputs=/*
  Product{,1..3} (4 alike) : Product
  Sum : Sum  Inputs=-+
  Sum1 : Sum
  Terminator : Terminator
  alpha_aero_dot : Outport
  wires:
  Vel_U_V_W_dot_BUS/1 -> Bus Selector2/1
  Sum/1 -> Divide/2
  Divide/1 -> alpha_aero_dot/1  "alpha_dot_rad/s"
  Vel_U_V_W_BUS/1 -> Bus Selector3/1
  Bus Selector3/1 -> Product3/1, Product3/2, Product/1  "<U>"
  Bus Selector2/2 -> Product/2  "<W_dot>"
  Product/1 -> Sum/2
  Bus Selector3/2 -> Product2/2, Product1/1, Product2/1  "<W>"
  Bus Selector2/1 -> Product1/2  "<U_dot>"
  Product1/1 -> Sum/1
  Product3/1 -> Sum1/1
  Product2/1 -> Sum1/2
  States_BUS/1 -> Terminator/1
  Sum1/1 -> Divide/1

== system Flight_Simulation/State_Integration_pure_simulink/Vel_aero_dot_Calculation/beta_aero_dot ==
  States_BUS : Inport
  Vel_U_V_W_BUS : Inport  Port=2
  Vel_U_V_W_dot_BUS : Inport  Port=3
  V_aero_total_dot : Inport  Port=4
  Add : Sum  Inputs=+-
  Bus Selector : BusSelector  OutputSignals=Vel_aero_V_alpha_beta
  Bus Selector1 : BusSelector  OutputSignals=v_m/s,beta_rad
  Bus Selector2 : BusSelector  OutputSignals=V_dot
  Bus Selector3 : BusSelector  OutputSignals=V
  Divide : Product  Inputs=/*
  Product1 : Product  Inputs=3
  Product3 : Product
  Product4 : Product
  Trigonometric Function : Trigonometry  Operator=cos
  beta_aero_dot : Outport
  wires:
  Vel_U_V_W_dot_BUS/1 -> Bus Selector2/1
  Bus Selector1/1 -> Product3/1, Product1/2, Product1/1  "<v_m/s>"
  States_BUS/1 -> Bus Selector/1
  Divide/1 -> beta_aero_dot/1  "beta_dot_rad/s"
  Bus Selector/1 -> Bus Selector1/1  "<Vel_aero_V_alpha_beta>"
  Vel_U_V_W_BUS/1 -> Bus Selector3/1
  Bus Selector1/2 -> Trigonometric Function/1  "<beta_rad>"
  Bus Selector2/1 -> Product3/2  "<V_dot>"
  Bus Selector3/1 -> Product4/1  "<V>"
  V_aero_total_dot/1 -> Product4/2
  Product3/1 -> Add/1
  Product4/1 -> Add/2
  Add/1 -> Divide/2
  Trigonometric Function/1 -> Product1/3
  Product1/1 -> Divide/1

== system Flight_Simulation/Environment_Subsystems/Wind_Model/Gust_model_(1-cos)/Distance traveled through the gust ==
  v_m/s : Inport
  gust_flgs : Inport  Port=2
  Integrator : Integrator  ExternalReset=rising
  Product : Product
  distance_traveled : Outport
  wires:
  v_m/s/1 -> Product/1
  Product/1 -> Integrator/1
  Integrator/1 -> distance_traveled/1  "xyz_traveled_m"
  gust_flgs/1 -> Integrator/2, Product/2  "gust_flgs"

== system Flight_Simulation/Environment_Subsystems/Wind_Model/Gust_model_(1-cos)/Gust parameters ==
  Atmosphere_BUS : Inport
  F_g : Inport  Port=2
  altitude : Inport  Port=3
  Bus Selector : BusSelector  OutputSignals=rho_kg/m^3
  Divide : Product  Inputs=*/
  EAS2TAS : Product
  Square Root : Sqrt  SaturateOnIntegerOverflow=on
  Switch1 : Switch  Criteria=u2 > Threshold
  density at sea level : Constant  Value=Environment.Const.rho0
  gust_amplitude_CS-25 : MATLAB Function  TreatAsAtomicUnit=on
  gust_gradientlength : Constant  Value=Environment.gust.gradientlength
  gust_man_amplitude : Constant  Value=Environment.gust.man_amplitude
  gust_switch_auto : Constant  Value=Environment.gust.switch_auto
  gust_gradient_length : Outport
  gust_amplitudes : Outport  Port=2
  wires:
  EAS2TAS/1 -> Switch1/1  "gust_amplitudes_m/s"
  altitude/1 -> gust_amplitude_CS-25/2(h)
  gust_gradientlength/1 -> gust_gradient_length/1, gust_amplitude_CS-25/1(H)  "gust_gradient_length_m"
  Switch1/1 -> gust_amplitudes/1
  gust_switch_auto/1 -> Switch1/2
  gust_man_amplitude/1 -> Switch1/3  "gust_amplitudes_m/s"
  F_g/1 -> gust_amplitude_CS-25/3(Aircraft_Fg)
  Atmosphere_BUS/1 -> Bus Selector/1
  density at sea level/1 -> Divide/1
  Bus Selector/1 -> Divide/2  "<rho_kg/m^3>"
  Divide/1 -> Square Root/1
  Square Root/1 -> EAS2TAS/2
  gust_amplitude_CS-25/1(U_ds) -> EAS2TAS/1  "gust_amplitudes_m/s"

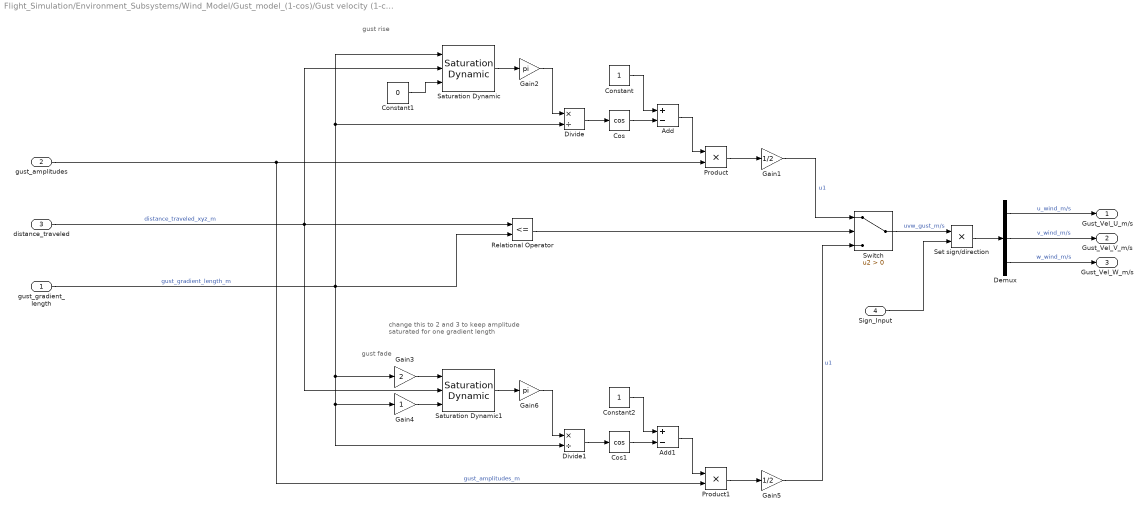
== system Flight_Simulation/Environment_Subsystems/Wind_Model/Gust_model_(1-cos)/Gust velocity (1-cos) ==
  note: change this to 2 and 3 to keep amplitude
      | saturated for one gradient length
  note: gust fade
  note: gust rise
  gust_gradient_length : Inport
  gust_amplitudes : Inport  Port=2
  distance_traveled : Inport  Port=3
  Sign_Input : Inport  Port=4
  Add : Sum  Inputs=+-
  Add1 : Sum  Inputs=+-
  Constant : Constant
  Constant1 : Constant  Value=0
  Constant2 : Constant
  Cos : Trigonometry  Operator=cos
  Cos1 : Trigonometry  Operator=cos
  Demux : Demux  Outputs=3
  Divide : Product  Inputs=*/
  Divide1 : Product  Inputs=*/
  Gain1 : Gain  Gain=1/2
  Gain2 : Gain  Gain=pi
  Gain3 : Gain  Gain=2
  Gain4 : Gain
  Gain5 : Gain  Gain=1/2
  Gain6 : Gain  Gain=pi
  Product : Product
  Product1 : Product
  Relational Operator : RelationalOperator  Operator=<=  OutDataTypeStr=boolean  RndMeth=Simplest
  Saturation Dynamic : simulink/Discontinuities/Saturation Dynamic  OutMin=[]  OutMax=[]  OutDataTypeStr=Inherit: Same as second input  OutDataType=fixdt(1, 16)  OutScaling=2^-10  DoSatur=off
  Saturation Dynamic1 : simulink/Discontinuities/Saturation Dynamic  OutMin=[]  OutMax=[]  OutDataTypeStr=Inherit: Same as second input  OutDataType=fixdt(1, 16)  OutScaling=2^-10  DoSatur=off
  Set sign/direction : Product
  Switch : Switch  Criteria=u2 > Threshold
  Gust_Vel_U_m/s : Outport
  Gust_Vel_V_m/s : Outport  Port=2
  Gust_Vel_W_m/s : Outport  Port=3
  wires:
  Relational Operator/1 -> Switch/2
  gust_gradient_length/1 -> Divide/2, Saturation Dynamic/1, Relational Operator/2, Divide1/2, Gain4/1, Gain3/1  "gust_gradient_length_m"
  distance_traveled/1 -> Relational Operator/1, Saturation Dynamic1/2, Saturation Dynamic/2  "distance_traveled_xyz_m"
  gust_amplitudes/1 -> Product1/2, Product/2  "gust_amplitudes_m"
  Constant1/1 -> Saturation Dynamic/3
  Constant/1 -> Add/1
  Add/1 -> Product/1
  Gain2/1 -> Divide/1
  Saturation Dynamic/1 -> Gain2/1
  Gain1/1 -> Switch/1  "u1"
  Divide/1 -> Cos/1
  Product/1 -> Gain1/1
  Cos/1 -> Add/2
  Gain4/1 -> Saturation Dynamic1/3
  Gain3/1 -> Saturation Dynamic1/1
  Constant2/1 -> Add1/1
  Add1/1 -> Product1/1
  Gain6/1 -> Divide1/1
  Saturation Dynamic1/1 -> Gain6/1
  Gain5/1 -> Switch/3  "u1"
  Divide1/1 -> Cos1/1
  Product1/1 -> Gain5/1
  Cos1/1 -> Add1/2
  Switch/1 -> Set sign/direction/1  "uvw_gust_m/s"
  Demux/2 -> Gust_Vel_V_m/s/1  "v_wind_m/s"
  Demux/1 -> Gust_Vel_U_m/s/1  "u_wind_m/s"
  Demux/3 -> Gust_Vel_W_m/s/1  "w_wind_m/s"
  Set sign/direction/1 -> Demux/1
  Sign_Input/1 -> Set sign/direction/2

== system Flight_Simulation/Environment_Subsystems/Wind_Model/Gust_model_(1-cos)/reset flags after gust ==
  note: delay necessary for triggered subsystem in a loop
  gust_u : Inport
  gust_v : Inport  Port=2
  gust_w : Inport  Port=3
  Abs : Abs
  Abs1 : Abs
  Abs2 : Abs
  Compare To Constant : simulink/Logic and Bit Operations/Compare To Constant  relop=>  const=0  OutDataTypeStr=boolean
  Compare To Constant1 : simulink/Logic and Bit Operations/Compare To Constant  relop=>  const=0  OutDataTypeStr=boolean
  Compare To Constant2 : simulink/Logic and Bit Operations/Compare To Constant  relop=>  const=0  OutDataTypeStr=boolean
  Detect Decrease : simulink/Logic and Bit Operations/Detect Decrease  vinit=0.0  OutDataTypeStr=boolean
  Detect Decrease1 : simulink/Logic and Bit Operations/Detect Decrease  vinit=0.0  OutDataTypeStr=boolean
  Detect Decrease2 : simulink/Logic and Bit Operations/Detect Decrease  vinit=0.0  OutDataTypeStr=boolean
  Mux : Mux  Inputs=3
  Triggered Subsystem : Subsystem  TreatAsAtomicUnit=on
  Triggered Subsystem1 : Subsystem  TreatAsAtomicUnit=on
  Triggered Subsystem2 : Subsystem  TreatAsAtomicUnit=on
  Unit Delay : UnitDelay  SampleTime=-1  HasFrameUpgradeWarning=on
  Unit Delay1 : UnitDelay  SampleTime=-1  HasFrameUpgradeWarning=on
  Unit Delay2 : UnitDelay  SampleTime=-1  HasFrameUpgradeWarning=on
  reset_flgs : Outport
  wires:
  Detect Decrease/1 -> Unit Delay/1
  gust_v/1 -> Abs2/1
  gust_w/1 -> Abs1/1
  Compare To Constant/1 -> Detect Decrease/1
  Triggered Subsystem2/1(w_flg) -> Mux/3  "reset_flg_w"
  gust_u/1 -> Abs/1
  Triggered Subsystem1/1(v_flg) -> Mux/2  "reset_flg_v"
  Triggered Subsystem/1(u_flg) -> Mux/1  "reset_flg_u"
  Detect Decrease1/1 -> Unit Delay1/1
  Detect Decrease2/1 -> Unit Delay2/1
  Compare To Constant2/1 -> Detect Decrease2/1
  Compare To Constant1/1 -> Detect Decrease1/1
  Unit Delay/1 -> Triggered Subsystem/Trigger
  Unit Delay1/1 -> Triggered Subsystem1/Trigger
  Unit Delay2/1 -> Triggered Subsystem2/Trigger
  Abs/1 -> Compare To Constant/1
  Abs1/1 -> Compare To Constant2/1
  Abs2/1 -> Compare To Constant1/1
  Mux/1 -> reset_flgs/1

== system Flight_Simulation/Non-linear_Plant/6DOF_Equations/Acceleration_nx_ny_nz_Calculation/nx_cg ==
  States_BUS : Inport
  Vel_U_V_W_dot_BUS : Inport  Port=2
  Gravity : Inport  Port=3
  Add : Sum  Inputs=-++
  Add1 : Sum
  Bus Selector : BusSelector  OutputSignals=Angles_phi_theta_psi
  Bus Selector1 : BusSelector  OutputSignals=theta_rad
  Bus Selector2 : BusSelector  OutputSignals=Rates_p_q_r
  Bus Selector3 : BusSelector  OutputSignals=q_rad/s,r_rad/s
  Bus Selector4 : BusSelector  OutputSignals=U_dot
  Bus Selector5 : BusSelector  OutputSignals=V_m/s,W_m/s
  Bus Selector6 : BusSelector  OutputSignals=Vel_U_V_W_body
  Constant : Constant
  Divide : Product  Inputs=/*
  Divide1 : Product
  Product : Product
  Product1 : Product
  Trigonometric Function : Trigonometry
  n_x_cg : Outport
  wires:
  Add1/1 -> n_x_cg/1  "n_x_cg"
  Constant/1 -> Divide/2
  Gravity/1 -> Divide/1
  States_BUS/1 -> Bus Selector/1, Bus Selector6/1, Bus Selector2/1
  Bus Selector/1 -> Bus Selector1/1  "<Angles_phi_theta_psi>"
  Bus Selector1/1 -> Trigonometric Function/1  "<theta_rad>"
  Bus Selector2/1 -> Bus Selector3/1  "<Rates_p_q_r>"
  Vel_U_V_W_dot_BUS/1 -> Bus Selector4/1
  Bus Selector4/1 -> Add/3  "<U_dot>"
  Bus Selector3/2 -> Product1/1  "<r_rad/s>"
  Bus Selector3/1 -> Product/1  "<q_rad/s>"
  Bus Selector5/2 -> Product/2  "<W_m/s>"
  Product/1 -> Add/2
  Bus Selector5/1 -> Product1/2  "<V_m/s>"
  Product1/1 -> Add/1
  Add/1 -> Divide1/1
  Divide/1 -> Divide1/2
  Divide1/1 -> Add1/2
  Trigonometric Function/1 -> Add1/1
  Bus Selector6/1 -> Bus Selector5/1  "<Vel_U_V_W_body>"

== system Flight_Simulation/Non-linear_Plant/6DOF_Equations/Acceleration_nx_ny_nz_Calculation/ny_cg ==
  States_BUS : Inport
  Vel_U_V_W_dot_BUS : Inport  Port=2
  Gravity : Inport  Port=3
  Add : Sum  Inputs=+-+
  Add1 : Sum  Inputs=-+
  Bus Selector : BusSelector  OutputSignals=Angles_phi_theta_psi
  Bus Selector1 : BusSelector  OutputSignals=phi_rad,theta_rad
  Bus Selector2 : BusSelector  OutputSignals=Rates_p_q_r
  Bus Selector3 : BusSelector  OutputSignals=p_rad/s,r_rad/s
  Bus Selector4 : BusSelector  OutputSignals=V_dot
  Bus Selector5 : BusSelector  OutputSignals=U_m/s,W_m/s
  Bus Selector6 : BusSelector  OutputSignals=Vel_U_V_W_body
  Constant : Constant
  Divide : Product  Inputs=/*
  Divide1 : Product
  Divide2 : Product
  Product : Product
  Product1 : Product
  Trigonometric Function : Trigonometry  Operator=cos
  Trigonometric Function1 : Trigonometry
  n_y_cg : Outport
  wires:
  Divide2/1 -> Add1/1
  Divide1/1 -> Add1/2
  Divide/1 -> Divide1/2
  Add/1 -> Divide1/1
  Product1/1 -> Add/1
  Bus Selector5/1 -> Product1/2  "<U_m/s>"
  Product/1 -> Add/2
  Bus Selector5/2 -> Product/2  "<W_m/s>"
  Bus Selector3/1 -> Product/1  "<p_rad/s>"
  Bus Selector3/2 -> Product1/1  "<r_rad/s>"
  Bus Selector4/1 -> Add/3  "<V_dot>"
  Vel_U_V_W_dot_BUS/1 -> Bus Selector4/1
  Bus Selector2/1 -> Bus Selector3/1  "<Rates_p_q_r>"
  Bus Selector1/2 -> Trigonometric Function/1  "<theta_rad>"
  Bus Selector/1 -> Bus Selector1/1  "<Angles_phi_theta_psi>"
  States_BUS/1 -> Bus Selector6/1, Bus Selector2/1, Bus Selector/1
  Gravity/1 -> Divide/1
  Constant/1 -> Divide/2
  Add1/1 -> n_y_cg/1  "n_y_cg"
  Bus Selector1/1 -> Trigonometric Function1/1  "<phi_rad>"
  Trigonometric Function/1 -> Divide2/2
  Trigonometric Function1/1 -> Divide2/1
  Bus Selector6/1 -> Bus Selector5/1  "<Vel_U_V_W_body>"

== system Flight_Simulation/Non-linear_Plant/6DOF_Equations/Acceleration_nx_ny_nz_Calculation/nz_cg ==
  States_BUS : Inport
  Vel_U_V_W_dot_BUS : Inport  Port=2
  Gravity : Inport  Port=3
  Add : Sum  Inputs=-++
  Add1 : Sum
  Bus Selector : BusSelector  OutputSignals=Angles_phi_theta_psi
  Bus Selector1 : BusSelector  OutputSignals=phi_rad,theta_rad
  Bus Selector2 : BusSelector  OutputSignals=Rates_p_q_r
  Bus Selector3 : BusSelector  OutputSignals=p_rad/s,q_rad/s
  Bus Selector4 : BusSelector  OutputSignals=W_dot
  Bus Selector5 : BusSelector  OutputSignals=U_m/s,V_m/s
  Bus Selector6 : BusSelector  OutputSignals=Vel_U_V_W_body
  Constant : Constant  Value=-1
  Divide : Product  Inputs=/*
  Divide1 : Product
  Divide2 : Product
  Product : Product
  Product1 : Product
  Trigonometric Function : Trigonometry  Operator=cos
  Trigonometric Function1 : Trigonometry  Operator=cos
  n_z_cg : Outport
  wires:
  Divide2/1 -> Add1/1
  Divide1/1 -> Add1/2
  Divide/1 -> Divide1/2
  Add/1 -> Divide1/1
  Product1/1 -> Add/1  "QU"
  Bus Selector5/1 -> Product1/2  "<U_m/s>"
  Product/1 -> Add/2  "PV"
  Bus Selector5/2 -> Product/2  "<V_m/s>"
  Bus Selector3/1 -> Product/1  "<p_rad/s>"
  Bus Selector3/2 -> Product1/1  "<q_rad/s>"
  Bus Selector4/1 -> Add/3  "<W_dot>"
  Vel_U_V_W_dot_BUS/1 -> Bus Selector4/1
  Bus Selector2/1 -> Bus Selector3/1  "<Rates_p_q_r>"
  Bus Selector1/2 -> Trigonometric Function/1  "<theta_rad>"
  Bus Selector/1 -> Bus Selector1/1  "<Angles_phi_theta_psi>"
  States_BUS/1 -> Bus Selector6/1, Bus Selector2/1, Bus Selector/1
  Gravity/1 -> Divide/1
  Constant/1 -> Divide/2
  Add1/1 -> n_z_cg/1  "n_z_cg"
  Bus Selector1/1 -> Trigonometric Function1/1  "<phi_rad>"
  Trigonometric Function/1 -> Divide2/2
  Trigonometric Function1/1 -> Divide2/1
  Bus Selector6/1 -> Bus Selector5/1  "<Vel_U_V_W_body>"

== system Flight_Simulation/Non-linear_Plant/6DOF_Equations/Attitude_Differential_Equations/phi_dot ==
  phi : Inport
  theta : Inport  Port=2
  psi : Inport  Port=3
  p : Inport  Port=4
  q : Inport  Port=5
  r : Inport  Port=6
  Product : Product
  Product1 : Product
  Product2 : Product
  Sum : Sum
  Sum1 : Sum
  Terminator : Terminator
  Trigonometric Function : Trigonometry
  Trigonometric Function3 : Trigonometry  Operator=cos
  Trigonometric Function7 : Trigonometry  Operator=tan
  phi_dot_rad/s : Outport
  wires:
  Sum/1 -> Product2/2
  Sum1/1 -> phi_dot_rad/s/1  "phi_dot_rad/s"
  r/1 -> Product1/2
  Trigonometric Function7/1 -> Product2/1
  Product/1 -> Sum/1
  Trigonometric Function/1 -> Product/1
  Trigonometric Function3/1 -> Product1/1
  p/1 -> Sum1/1
  Product2/1 -> Sum1/2
  q/1 -> Product/2
  Product1/1 -> Sum/2
  theta/1 -> Trigonometric Function7/1
  phi/1 -> Trigonometric Function/1, Trigonometric Function3/1
  psi/1 -> Terminator/1

== system Flight_Simulation/Non-linear_Plant/6DOF_Equations/Attitude_Differential_Equations/psi_dot ==
  phi : Inport
  theta : Inport  Port=2
  psi : Inport  Port=3
  p : Inport  Port=4
  q : Inport  Port=5
  r : Inport  Port=6
  Divide : Product  Inputs=/*
  Product : Product
  Product1 : Product
  Sum : Sum
  Terminator : Terminator
  Terminator2 : Terminator
  Trigonometric Function : Trigonometry
  Trigonometric Function1 : Trigonometry  Operator=cos
  Trigonometric Function3 : Trigonometry  Operator=cos
  psi_dot_rad/s : Outport
  wires:
  p/1 -> Terminator/1
  Divide/1 -> psi_dot_rad/s/1  "psi_dot_rad/s"
  r/1 -> Product1/2
  q/1 -> Product/2
  Product/1 -> Sum/1
  Product1/1 -> Sum/2
  theta/1 -> Trigonometric Function1/1
  psi/1 -> Terminator2/1
  phi/1 -> Trigonometric Function3/1, Trigonometric Function/1
  Trigonometric Function1/1 -> Divide/1
  Sum/1 -> Divide/2  "psi_dot_rad/s"
  Trigonometric Function/1 -> Product/1
  Trigonometric Function3/1 -> Product1/1

== system Flight_Simulation/Non-linear_Plant/6DOF_Equations/Attitude_Differential_Equations/theta_dot ==
  phi : Inport
  theta : Inport  Port=2
  psi : Inport  Port=3
  p : Inport  Port=4
  q : Inport  Port=5
  r : Inport  Port=6
  Product : Product
  Product1 : Product
  Sum : Sum  Inputs=+-
  Terminator : Terminator
  Terminator1 : Terminator
  Terminator2 : Terminator
  Trigonometric Function : Trigonometry
  Trigonometric Function3 : Trigonometry  Operator=cos
  theta_dot_rad/s : Outport
  wires:
  phi/1 -> Trigonometric Function/1, Trigonometric Function3/1
  psi/1 -> Terminator2/1
  theta/1 -> Terminator1/1
  Product1/1 -> Sum/2
  Product/1 -> Sum/1
  Trigonometric Function3/1 -> Product/1
  q/1 -> Product/2
  r/1 -> Product1/2
  Trigonometric Function/1 -> Product1/1
  Sum/1 -> theta_dot_rad/s/1  "theta_dot_rad/s"
  p/1 -> Terminator/1

== system Flight_Simulation/Non-linear_Plant/6DOF_Equations/Position_Differential_Equations/Calculate_alt_position_dot1 ==
  U : Inport
  V : Inport  Port=2
  W : Inport  Port=3
  phi : Inport  Port=4
  theta : Inport  Port=5
  psi : Inport  Port=6
  Product : Product
  Product1 : Product  Inputs=3
  Product2 : Product  Inputs=3
  Sum2 : Sum  Inputs=+--
  Terminator : Terminator
  Terminator1 : Terminator
  Trigonometric Function4 : Trigonometry  Operator=cos
  Trigonometric Function5 : Trigonometry  Operator=cos
  Trigonometric Function6 : Trigonometry
  Trigonometric Function7 : Trigonometry
  Trigonometric Function8 : Trigonometry  Operator=cos
  Trigonometric Function9 : Trigonometry
  alt_dot : Outport
  wires:
  phi/1 -> Trigonometric Function6/1, Trigonometric Function5/1
  psi/1 -> Trigonometric Function9/1, Trigonometric Function8/1
  theta/1 -> Trigonometric Function7/1, Trigonometric Function4/1
  Sum2/1 -> alt_dot/1  "alt_dot_m/s"
  U/1 -> Product/1
  Trigonometric Function7/1 -> Product/2
  V/1 -> Product1/1
  Trigonometric Function6/1 -> Product1/2
  Trigonometric Function4/1 -> Product2/3, Product1/3
  Product/1 -> Sum2/1
  Product1/1 -> Sum2/2
  W/1 -> Product2/1
  Trigonometric Function5/1 -> Product2/2
  Trigonometric Function8/1 -> Terminator/1
  Trigonometric Function9/1 -> Terminator1/1
  Product2/1 -> Sum2/3

== system Flight_Simulation/Non-linear_Plant/6DOF_Equations/Position_Differential_Equations/Calculate_east_position_dot ==
  U : Inport
  V : Inport  Port=2
  W : Inport  Port=3
  phi : Inport  Port=4
  theta : Inport  Port=5
  psi : Inport  Port=6
  Product3 : Product  Inputs=3
  Product4 : Product  Inputs=3
  Product{5..6,8..9} (4 alike) : Product
  Product7 : Product  Inputs=3
  Sum : Sum
  Sum1 : Sum  Inputs=+-
  Sum2 : Sum  Inputs=+++
  Trigonometric Function4 : Trigonometry  Operator=cos
  Trigonometric Function5 : Trigonometry  Operator=cos
  Trigonometric Function6 : Trigonometry
  Trigonometric Function7 : Trigonometry
  Trigonometric Function8 : Trigonometry  Operator=cos
  Trigonometric Function9 : Trigonometry
  east_pos_dot : Outport
  wires:
  Product8/1 -> Sum1/2
  Product6/1 -> Sum2/2
  Sum2/1 -> east_pos_dot/1  "east_pos_dot_m/s"
  Product9/1 -> Sum2/3
  Product4/1 -> Sum/1
  Sum1/1 -> Product9/2
  theta/1 -> Trigonometric Function4/1, Trigonometric Function7/1
  Product7/1 -> Sum1/1
  Sum/1 -> Product6/2
  Product3/1 -> Sum2/1
  psi/1 -> Trigonometric Function8/1, Trigonometric Function9/1
  Product5/1 -> Sum/2
  phi/1 -> Trigonometric Function5/1, Trigonometric Function6/1
  U/1 -> Product3/1
  Trigonometric Function4/1 -> Product3/2
  Trigonometric Function9/1 -> Product7/3, Product4/2, Product3/3
  V/1 -> Product6/1
  Trigonometric Function6/1 -> Product8/1, Product4/1
  Trigonometric Function7/1 -> Product7/2, Product4/3
  Trigonometric Function5/1 -> Product7/1, Product5/1
  Trigonometric Function8/1 -> Product8/2, Product5/2
  W/1 -> Product9/1
